simulink model "flexcan_can_fd_slave_s32k14"  (R2017a)
settings: Solver=FixedStepDiscrete  StartTime=0.0  StopTime=10.0  FixedStep=0.1  RelTol=1e-3  EnableMultiTasking=on
InitFcn:
  | mbd_s32k14_consistency_checks(bdroot(gcs));
model workspace (MAT data in the model file):
  MCOS : class17 (value not decoded)
undefined symbols (not defined in the file): A10, AD12, AD6, AD7, Aligned, B10, B8, B9, C10, C7, C8, C9, D1, D2, D8, Edge, External, G2, G3, G5, G6, H8, J8, K10, K5, K9, PTA1, PTA2, PTA3, PTB10, PTB11, PTB12, PTB8, PTB9, PTC10, PTC11, PTC12, PTC13, PTC14, PTC6, PTC7, PTD10, PTD11, PTD15, PTD16, PTD4, PTE4, PTE5, SpeedControllerIntegGain, SpeedControllerPropGain, TRGMUX_PDB_TRIG
libraries: mbd_s32k14_ec_toolbox x31, simulink x10
(part 2 of 2)

== system flexcan_can_fd_slave_s32k14/RX_Complete_Event/Function-Call Subsystem/Event_Control/ControlEventLogic/ToggleLED_HallA ==
  function : TriggerPort  TriggerType=function-call  VariantControl=Variant
  Data Store Read1 : DataStoreRead  DataStoreName=HallInputA
  Data Store Write1 : DataStoreWrite  DataStoreName=HallInputA
  Function-Call Generator : simulink/Ports & Subsystems/Function-Call Generator  sample_time=-1  numberOfIterations=1
  Logical Operator : Logic  Operator=NOT  AllPortsSameDT=off  OutDataTypeStr=boolean
  Call : Outport
  wires:
  Function-Call Generator/1 -> Call/1
  Data Store Read1/1 -> Logical Operator/1
  Logical Operator/1 -> Data Store Write1/1

== system flexcan_can_fd_slave_s32k14/RX_Complete_Event/Function-Call Subsystem/Event_Control/ControlEventLogic/ToggleLED_HallB ==
  function : TriggerPort  TriggerType=function-call  VariantControl=Variant
  Data Store Read1 : DataStoreRead  DataStoreName=HallInputB
  Data Store Write1 : DataStoreWrite  DataStoreName=HallInputB
  Function-Call Generator : simulink/Ports & Subsystems/Function-Call Generator  sample_time=-1  numberOfIterations=1
  Logical Operator : Logic  Operator=NOT  AllPortsSameDT=off  OutDataTypeStr=boolean
  Call : Outport
  wires:
  Function-Call Generator/1 -> Call/1
  Data Store Read1/1 -> Logical Operator/1
  Logical Operator/1 -> Data Store Write1/1

== system flexcan_can_fd_slave_s32k14/RX_Complete_Event/Function-Call Subsystem/Event_Control/ControlEventLogic/ToggleLED_HallC ==
  function : TriggerPort  TriggerType=function-call  VariantControl=Variant
  Data Store Read1 : DataStoreRead  DataStoreName=HallInputC
  Data Store Write1 : DataStoreWrite  DataStoreName=HallInputC
  Function-Call Generator : simulink/Ports & Subsystems/Function-Call Generator  sample_time=-1  numberOfIterations=1
  Logical Operator : Logic  Operator=NOT  AllPortsSameDT=off  OutDataTypeStr=boolean
  Call : Outport
  wires:
  Function-Call Generator/1 -> Call/1
  Data Store Read1/1 -> Logical Operator/1
  Logical Operator/1 -> Data Store Write1/1

== stateflow chart flexcan_can_fd_slave_s32k14/RX_Complete_Event/SwitchFunction/Chart ==
  state SwitchCheck1 [parallel]
    settings: executionOrder=1
    state Decrement
      du:out = 0;
      (default) -> (junction 19)
      Decrement -> (junction 19) [order 1] : [((Increment ==0)& ...
          |  (Decrement==1))& hasChanged(Increment)]
          | {out=1000;}
    state Increment
      du:out = 0;
      (default) -> (junction 11)
      Increment -> (junction 11) [order 1] : [((Increment ==1)& ...
          |  (Decrement==0))&hasChanged(Decrement)]
          | {out=0;}
    (default) -> Decrement : { out =0;}
    Increment -> Decrement [order 1] : [(Increment==0)& ...
        |  (Decrement==1) ...
        | & hasChanged(Increment)]
        | {out=-100;}
    Decrement -> Increment [order 1] : [((Increment ==1)& ...
        |  (Decrement==0))&hasChanged(Decrement)]
        | {out=100;}
  data: out output int16; Increment input boolean; Decrement input boolean

== stateflow chart flexcan_can_fd_slave_s32k14/RX_Complete_Event/Switch Case Action Subsystem ID_0x3FF/Chart ==
  state A
  state A1
  (default) -> A
  A -> A1
  A1 -> A
  data: A output boolean [0..1]

== stateflow chart flexcan_can_fd_slave_s32k14/RX_Complete_Event/Function-Call Subsystem/CalculateRPM/Actual Motor Speed Calculation/GatherNumberOfHallStateChanges ==
  (default) -> (junction 5)
  (junction 5) -> (junction 6) : {
      | 	HallChangesSum = HallChangesSum - StoreHallChanges[i];
      | 	StoreHallChanges[i] = HallChanges;
      | 	HallChangesSum = HallChangesSum + StoreHallChanges[i];
      | 	i++;
      | }
  (junction 6) -> (junction 22) [order 2] : {
      | 	HallChangeClear = 0;
      | }
  (junction 6) -> (junction 6) [order 1] : [i >= 250]
      | {i=0;}
  data: StoreHallChanges local uint8 size=[250]; HallChanges input; HallChangesSum output uint16; i local uint8; HallChangeClear output

== stateflow chart flexcan_can_fd_slave_s32k14/RX_Complete_Event/Function-Call Subsystem/Event_Control/ControlPollingLogic ==
  state Logic1
    Logic1 -> (junction 25)
    (default) -> (junction 25)
    (junction 25) -> (junction 26) [order 1] : [(MotorSpeedRPM <= 100) && (MotorSpeedRPM >= -100)]
        | {Trigger;}
    (junction 25) -> (junction 28) [order 2]
    (junction 26) -> (junction 27)
    (junction 28) -> (junction 27)
  (default) -> Logic1
  data: MotorSpeedRPM input
  events: Trigger output FUNCTION_CALL_EVENT

== stateflow chart flexcan_can_fd_slave_s32k14/RX_Complete_Event/Function-Call Subsystem/Control_Logic/FET pre-driver Initialization Sequence ==
  settings: sampleTime=0.500
  state A
  state B
  state C
  state C1
  state C2
  state D
  state E
  state F
    F -> F [order 1] : {index++;}
  state END
  (default) -> A : {enable=0;}
  A -> B : /*MASK0*/
      | {MPC_Data = 0x20;}
  B -> C : /*MASK1*/
      | {MPC_Data = 0x30;}
  C -> C1 : /*CLINT0*/
      | {MPC_Data = 0x6F;}
  C1 -> C2 : /*CLINT1*/
      | {MPC_Data = 0x7F;}
  C2 -> D : /*Mode*/
      | {MPC_Data  = 0x48;}
  D -> E : {MPC_Data = 0x00;
      | enable=1;}
  E -> F : {Charge_Bootstrap_Low_On;
      | index=0;}
  F -> END [order 1] : [index > 0]
      | {Charge_Bootstrap_All_Off;}
  END -> END : {Normal_Op;
      | MPC_Data = MPC_Cmd;}
  data: MPC_Data output uint16; enable output boolean; index local double; MPC_Cmd data_store_memory
  events: Charge_Bootstrap_Low_On output FUNCTION_CALL_EVENT; Charge_Bootstrap_All_Off output FUNCTION_CALL_EVENT; Normal_Op output FUNCTION_CALL_EVENT

== stateflow chart flexcan_can_fd_slave_s32k14/RX_Complete_Event/If Action Subsystem/If Action Subsystem/Chart ==
  state SwitchCheck1 [parallel]
    settings: executionOrder=1
    state Decrement
      du:out = 0;
      (default) -> (junction 19)
      Decrement -> (junction 19) [order 1] : [((Increment ==0)& ...
          |  (Decrement==1))& hasChanged(Increment)]
          | {out=100;}
    state Increment
      du:out = 0;
      (default) -> (junction 11)
      Increment -> (junction 11) [order 1] : [((Increment ==1)& ...
          |  (Decrement==0))&hasChanged(Decrement)]
          | {out=-100;}
    (default) -> Decrement : { out =0;}
    Increment -> Decrement [order 1] : [(Increment==0)& ...
        |  (Decrement==1) ...
        | & hasChanged(Increment)]
        | {out=-100;}
    Decrement -> Increment [order 1] : [((Increment ==1)& ...
        |  (Decrement==0))&hasChanged(Decrement)]
        | {out=100;}
  data: out output int16; Increment input boolean; Decrement input boolean

== stateflow chart flexcan_can_fd_slave_s32k14/RX_Complete_Event/Function-Call Subsystem/Event_Control/Init ==
  settings: sampleTime=0.500
  state A
  state B
  (default) -> A
  A -> B : {Init;
      | index=0;}
  B -> B
  data: index local double
  events: Init output FUNCTION_CALL_EVENT

== stateflow chart flexcan_can_fd_slave_s32k14/RX_Complete_Event/Function-Call Subsystem/Trapezoidal_Commutation/CommutationTableLookup ==
  (junction 5) -> (junction 15) [order 1] : /*If Direction is Negative */
      | [Direction == -1]
  (default) -> (junction 5)
  (junction 15) -> (junction 14) : {
      |    Phase_A = ccwTable[HallState][0];
      |    Phase_B = ccwTable[HallState][1];
      |    Phase_C = ccwTable[HallState][2];
      | }
  (junction 5) -> (junction 6) [order 2] : {
      |    Phase_A = cwTable[HallState][0];
      |    Phase_B = cwTable[HallState][1];
      |    Phase_C = cwTable[HallState][2];
      | }
  (junction 6) -> (junction 14)
  data: cwTable constant uint8 size=[8 3] =[0 0 0; 2 1 0; 0 2 1; 2 0 1; 1 0 2; 0 1 2; 1 2 0; 0 0 0]; HallState input; Phase_A output uint8; Phase_B output uint8; Phase_C output uint8; ccwTable constant uint8 size=[8 3] =[0 0 0; 1 2 0; 0 1 2; 1 0 2; 2 0 1; 0 2 1; 2 1 0; 0 0 0]; Direction input

== stateflow chart flexcan_can_fd_slave_s32k14/RX_Complete_Event/Function-Call Subsystem/Trapezoidal_Commutation/PhaseSwitchLogic ==
  settings: sampleTime=0.500
  note: Phase States:
      | 0 = NC
      | 1 = -Vdcb
      | 2 = +Vdcb
  (default) -> (junction 13)
  (junction 13) -> (junction 14) [order 1] : /*check for phase state 0 */
      | [Phase_A == 0]
      | /*set output for state 0 */
      | {Phase_A_HS = 0; Phase_A_LS =0;}
  (junction 13) -> (junction 17) [order 2]
  (junction 14) -> (junction 16)
  (junction 17) -> (junction 16) [order 1] : /*check for phase state 1 */
      | [Phase_A == 1]
      | /*set output for state 1 */
      | {Phase_A_HS = 0; Phase_A_LS = PWM_Duty_Cycle;}
  (junction 17) -> (junction 20) [order 2]
  (junction 16) -> (junction 19)
  (junction 20) -> (junction 19) [order 1] : /*check for phase state 2 */
      | [Phase_A == 2]
      | /*set output for state 2 */
      | {Phase_A_HS = 1000; Phase_A_LS = 0;}
  (junction 20) -> (junction 62) [order 2]
  (junction 19) -> (junction 23)
  (junction 62) -> (junction 23)
  (junction 23) -> (junction 22) [order 1] : /*check for phase state 0 */
      | [Phase_B == 0]
      | /*set output for state 0 */
      | {Phase_B_HS = 0; Phase_B_LS = 0;}
  (junction 23) -> (junction 26) [order 2]
  (junction 22) -> (junction 25)
  (junction 26) -> (junction 25) [order 1] : /*check for phase state 1 */
      | [Phase_B == 1]
      | /*set output for state 1 */
      | {Phase_B_HS = 0; Phase_B_LS = PWM_Duty_Cycle;}
  (junction 26) -> (junction 29) [order 2]
  (junction 25) -> (junction 28)
  (junction 29) -> (junction 28) [order 1] : /*check for phase state 2 */
      | [Phase_B == 2]
      | /*set output for state 2 */
      | {Phase_B_HS = 1000; Phase_B_LS = 0;}
  (junction 29) -> (junction 65) [order 2]
  (junction 28) -> (junction 49)
  (junction 65) -> (junction 49)
  (junction 49) -> (junction 48) [order 1] : /*check for phase state 0 */
      | [Phase_C == 0]
      | /*set output for state 0 */
      | {Phase_C_HS = 0; Phase_C_LS = 0;}
  (junction 49) -> (junction 51) [order 2]
  (junction 48) -> (junction 50)
  (junction 51) -> (junction 50) [order 1] : /*check for phase state 1 */
      | [Phase_C == 1]
      | /*set output for state 1 */
      | {Phase_C_HS = 0; Phase_C_LS = PWM_Duty_Cycle;}
  (junction 51) -> (junction 53) [order 2]
  (junction 50) -> (junction 52)
  (junction 53) -> (junction 52) [order 1] : /*check for phase state 2 */
      | [Phase_C == 2]
      | /*set output for state 2 */
      | {Phase_C_HS = 1000; Phase_C_LS = 0;}
  (junction 53) -> (junction 70) [order 2]
  (junction 52) -> (junction 69)
  (junction 70) -> (junction 69)
  data: Phase_A input; Phase_B input; Phase_C input; Phase_A_HS output uint32; Phase_A_LS output uint32; Phase_B_HS output uint32; Phase_B_LS output uint32; Phase_C_HS output uint32; Phase_C_LS output uint32; PWM_Duty_Cycle input
